simulink model "Full_RC_with_AVO"  (Simulink 8.3)
settings: Solver=ode1  StartTime=0.0  StopTime=500000.0  FixedStep=0.1  RelTol=1e-3
libraries: simulink x2
settings Model: Creator=user  LastModifiedBy=user
settings DataIOCC: SignalLoggingSaveFormat=Dataset
settings DebuggingCC: UnderspecifiedInitializationDetection=Simplified  StateNameClashWarn=none
settings GRTTargetCC: CombineOutputUpdateFcns=on  GRTInterface=off

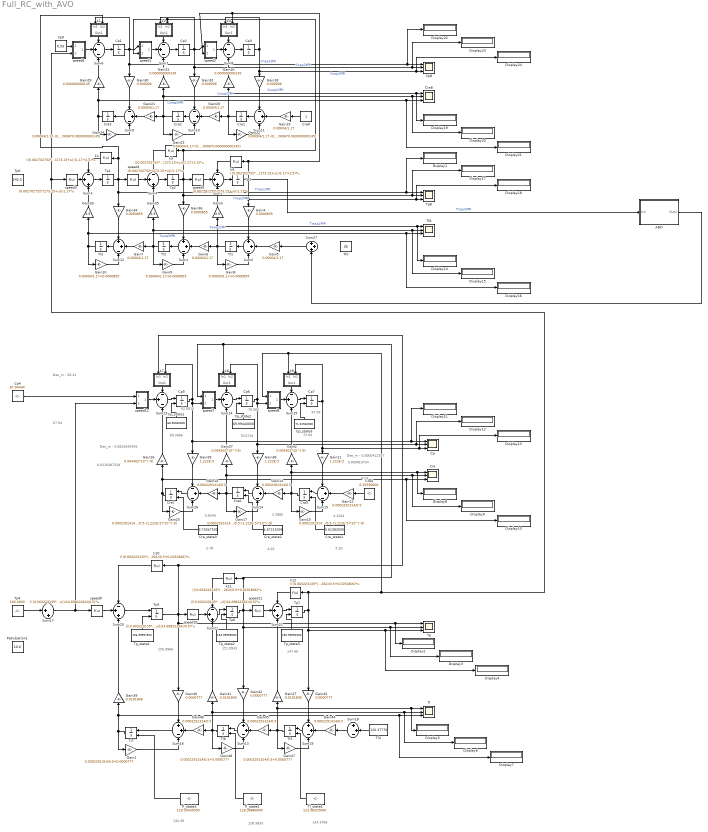
== system Full_RC_with_AVO ==
  note: Des_m - 0.0000412357
  note: Des_m - 0.0815645409
  note: 0.000010734
  note: 0.0216487318
  note: 0.9249
  note: 2.3980
  note: 4.2264
  note: 62.8910
  note: 78.085
  note: 97.09
  note: 67.94
  note: 2.78
  note: 4.02
  note: 5.26
  note: 72.04
  note: 70.6733
  note: 69.3066
  note: 132.39
  note: 128.3833
  note: 124.3766
  note: 147.99
  note: 151.9933
  note: 156.9966
  note: 4.24
  note: Des_m - 50.41
  Cp : Scope  NumInputPorts=3
      settings: TickLabels=on  ShowLegends=on  YMin=50~75~90  YMax=64~100~150  SaveName=CV_SM  DataFormat=Structure  SampleInput=on
  Cp0 : Constant  Value=0.53
  Cp1 : Integrator  InitialCondition=0.665
  Cp2 : Integrator  InitialCondition=0.803
  Cp3 : Integrator  InitialCondition=0.986
  Cp4 : Constant  Value=67.94440
  Cp5 : Integrator  InitialConditionSource=external  InitialCondition=69.3066
  Cp6 : Integrator  InitialConditionSource=external  InitialCondition=70.6733
  Cp7 : Integrator  InitialConditionSource=external  InitialCondition=72.04
  Cp8 : Scope  NumInputPorts=3
      settings: TickLabels=on  ShowLegends=on  YMin=50~75~90  YMax=64~100~150  SaveName=CV_SM1  DataFormat=Structure  SampleInput=on
  Cp_state1 : Constant  Value=68.96940000
  Cp_state2 : Constant  Value=69.99440000
  Cp_state3 : Constant  Value=71.01940000
  Cra : Scope  NumInputPorts=3
      settings: TickLabels=on  ShowLegends=on  YMin=4.17~2.4~0.84  YMax=4.28~2.5~1  SaveName=CF_SM  SampleInput=on
  Cra0 : Constant
  Cra1 : Integrator  InitialCondition=0.827
  Cra2 : Integrator  InitialCondition=0.6862
  Cra3 : Integrator  InitialCondition=0.5696
  Cra4 : Constant  Value=6.55550000
  Cra5 : Integrator  InitialConditionSource=external  InitialCondition=5.26
  Cra6 : Integrator  InitialConditionSource=external  InitialCondition=4.02
  Cra7 : Integrator  InitialConditionSource=external  InitialCondition=2.78
  Cra8 : Scope  NumInputPorts=3
      settings: TickLabels=on  ShowLegends=on  YMin=4.17~2.4~0.84  YMax=4.28~2.5~1  SaveName=CF_SM1  SampleInput=on
  Cra_state1 : Constant  Value=5.61382500
  Cra_state2 : Constant  Value=4.67215000
  Cra_state3 : Constant  Value=3.73047500
  Display{1..24} (24 alike) : Display
  Gain1 : Gain  Gain=0.0002291314/0.5+0.0000777
  Gain10 : Gain  Gain=0.00004/1.17+0.0000855
  Gain11 : Gain  Gain=1.222E-5
  Gain{12..14,44..46} (6 alike) : Gain  Gain=0.0002291314/0.5
  Gain15 : Gain  Gain=0.0002291314/0.5-(1.222E-5)*10^(-9)
  Gain16 : Gain  Gain=0.000000000145
  Gain17 : Gain  Gain=0.0002291314/0.5-(1.222E-5)*10^(-9)
  Gain18 : Gain  Gain=0.000006
  Gain{5..7,19..21} (6 alike) : Gain  Gain=0.00004/1.17
  Gain2 : Gain  Gain=0.004302*10^(-9)
  Gain22 : Gain  Gain=0.00004/1.17-(0.000006*0.000000000145)
  Gain23 : Gain  Gain=0.00004/1.17-(0.000006*0.000000000145)
  Gain24 : Gain  Gain=0.00004/1.17-(0.000006*0.000000000145)
  Gain25 : Gain  Gain=0.0002291314/0.5-(1.222E-5)*10^(-9)
  Gain26 : Gain  Gain=0.004302*10^(-9)
  Gain27 : Gain  Gain=0.0191806
  Gain28 : Gain  Gain=1.222E-5
  Gain29 : Gain  Gain=0.000000000145
  Gain3 : Gain  Gain=2.5
  Gain30 : Gain  Gain=0.000006
  Gain31 : Gain  Gain=0.000000000145
  Gain32 : Gain  Gain=0.000006
  Gain33 : Gain  Gain=2.5
  Gain34 : Gain  Gain=0.0000855
  Gain35 : Gain  Gain=2.5
  Gain36 : Gain  Gain=0.0000855
  Gain37 : Gain  Gain=0.004302*10^(-9)
  Gain38 : Gain  Gain=1.222E-5
  Gain39 : Gain  Gain=0.0191806
  Gain4 : Gain  Gain=0.0000855
  Gain40 : Gain  Gain=0.0000777
  Gain41 : Gain  Gain=0.0191806
  Gain42 : Gain  Gain=0.0000777
  Gain43 : Gain  Gain=0.0000777
  Gain47 : Gain  Gain=0.0002291314/0.5+0.0000777
  Gain48 : Gain  Gain=0.0002291314/0.5+0.0000777
  Gain8 : Gain  Gain=0.00004/1.17+0.0000855
  Gain9 : Gain  Gain=0.00004/1.17+0.0000855
  Petrubation1 : Constant  Value=10.0
  Sum{1..2,12..13,16,18..19} (7 alike) : Sum  Inputs=++-
  Sum{6..11,14..15,23..26} (12 alike) : Sum  Inputs=-+-
  Sum17 : Sum  Inputs=|++
  Sum{3..5,20..22} (6 alike) : Sum  Inputs=-++
  Sum27 : Sum  Inputs=+++
  Tl : Scope  NumInputPorts=3
      settings: TickLabels=on  ShowLegends=on  YMin=13~10~8.800000000000001  YMax=15.2~21~10.55  SaveName=TF_SM  SampleInput=on
  Tl0 : Constant  Value=30
  Tl1 : Integrator  InitialCondition=58.28
  Tl2 : Integrator  InitialCondition=86.23
  Tl3 : Integrator  InitialCondition=111.75
  Tl4 : Constant  Value=120.37770
  Tl5 : Integrator  InitialConditionSource=external  InitialCondition=124.3766
  Tl6 : Integrator  InitialConditionSource=external  InitialCondition=128.3833
  Tl7 : Integrator  InitialConditionSource=external  InitialCondition=132.39
  Tl8 : Scope  NumInputPorts=3
      settings: TickLabels=on  ShowLegends=on  YMin=13~10~8.800000000000001  YMax=15.2~21~10.55  SaveName=TF_SM1  SampleInput=on
  "Tl_state1 " : Constant  Value=123.38325000
  Tl_state2 : Constant  Value=126.38880000
  Tl_state3 : Constant  Value=129.39435000
  Tp : Scope  NumInputPorts=3
      settings: TickLabels=on  ShowLegends=on  YMin=155.5~145~146  YMax=158.5~152~154.5  SaveName=TV_SM  SampleInput=on
  Tp0 : Constant  Value=142.5
  Tp1 : Integrator  InitialCondition=121.956
  Tp2 : Integrator  InitialCondition=97.4
  Tp3 : Integrator  InitialCondition=69.6  IgnoreLimit=on
  Tp4 : Constant  Value=160.0000
  Tp5 : Integrator  InitialConditionSource=external  InitialCondition=156.9966
  Tp6 : Integrator  InitialConditionSource=external  InitialCondition=151.9933
  Tp7 : Integrator  InitialConditionSource=external  InitialCondition=147.99  IgnoreLimit=on
  Tp8 : Scope  NumInputPorts=3
      settings: TickLabels=on  ShowLegends=on  YMin=155.5~145~146  YMax=158.5~152~154.5  SaveName=TV_SM1  SampleInput=on
  Tp_state1 : Constant  Value=156.99997500
  Tp_state2 : Constant  Value=153.99995000
  Tp_state3 : Constant  Value=150.99992500
  k1 : Subsystem
  k10 : Fcn  Expr=(((0.003223135*(273+u))/24.69822264)/0.5+0.0191806)*u
  k11 : Fcn  Expr=(((0.003223135*(273+u))/24.69822264)/0.5+0.0191806)*u
  k12 : Fcn  Expr=(((0.003223135*(273+u))/24.69822264)/0.5+0.0191806)*u
  k2 : Subsystem
  k3 : Subsystem
  k4 : Fcn  Expr=((0.002702752*(273.15+u))/1.17+2.5)*u
  k5 : Fcn  Expr=((0.002702752*(273.15+u))/1.17+2.5)*u
  k6 : Fcn  Expr=((0.002702752*(273.15+u))/1.17+2.5)*u
  k7 : Subsystem
  k8 : Subsystem
  k9 : Subsystem
  speed1 : Subsystem
  speed10 : Fcn  Expr=(((0.003223135*(273+u))/24.69822264)/0.5)*u
  speed11 : Fcn  Expr=(((0.003223135*(273+u))/24.69822264)/0.5)*u
  speed12 : Subsystem
  speed2 : Subsystem
  speed3 : Fcn  Expr=(0.002702752*(273.15+u))/1.17*u
  speed4 : Fcn  Expr=(0.002702752*(273.15+u))/1.17*u
  speed5 : Fcn  Expr=(0.002702752*(273.15+u))/1.17*u
  speed6 : Subsystem
  speed7 : Subsystem
  speed8 : Subsystem
  speed9 : Fcn  Expr=(((0.003223135*(273+u))/24.69822264)/0.5)*u
  АВО : Subsystem
  wires:
  Sum6/1 -> Cp1/1
  speed1/1(Out1) -> Sum7/2
  Sum7/1 -> Cp2/1
  speed2/1(Out1) -> Sum8/2
  Sum8/1 -> Cp3/1
  Cp1/1 -> Cp8/1, Display22/1, Gain30/1, k1/1(In1), speed1/1(In1)  "Cпар1УРК"
  Cp2/1 -> Display23/1, Cp8/2, Gain32/1, speed2/1(In1), k2/1(In1)  "Cпар2УРК"
  Gain29/1 -> Sum6/3
  Cp3/1 -> Display24/1, Cp8/3, Gain18/1, k3/1(In1)  "Cпар3УРК"
  Gain31/1 -> Sum7/3
  Gain16/1 -> Sum8/3
  Gain30/1 -> Sum9/1
  Gain32/1 -> Sum10/1
  Gain18/1 -> Sum11/1
  Gain19/1 -> Sum11/2
  Sum11/1 -> Cra1/1
  Cra1/1 -> Gain22/1, Gain20/1, Display19/1, Cra8/1, Gain16/1  "Cжид1УРК"
  Gain20/1 -> Sum10/2
  Sum10/1 -> Cra2/1
  Cra2/1 -> Gain23/1, Gain21/1, Display20/1, Cra8/2, Gain31/1  "Cжид2УРК"
  Gain21/1 -> Sum9/2
  Sum9/1 -> Cra3/1
  Cra3/1 -> Gain24/1, Display21/1, Cra8/3, Gain29/1  "Cжид3УРК"
  Gain22/1 -> Sum11/3
  Gain23/1 -> Sum10/3
  Gain24/1 -> Sum9/3
  speed3/1 -> Sum3/2
  k4/1 -> Sum3/1
  Sum3/1 -> Tp1/1
  speed4/1 -> Sum4/2
  k5/1 -> Sum4/1
  Sum4/1 -> Tp2/1
  speed5/1 -> Sum5/2
  k6/1 -> Sum5/1
  Sum5/1 -> Tp3/1
  Tp1/1 -> Display1/1, Tp8/1, Gain34/1, k4/1, k1/2(In2), speed4/1  "Tпар1УРК"
  Gain33/1 -> Sum3/3
  Tp3/1 -> АВО/1(In1), Display18/1, Tp8/3, Gain4/1, k6/1, k3/2(In2), speed2/2(In2)  "Tпар3УРК"
  Gain35/1 -> Sum4/3
  Gain3/1 -> Sum5/3
  Gain34/1 -> Sum12/1
  Gain36/1 -> Sum1/1
  Gain4/1 -> Sum2/1
  Gain5/1 -> Sum2/2
  Sum2/1 -> Tl1/1
  Tl1/1 -> Gain8/1, Gain6/1, Display14/1, Tl8/1, Gain3/1  "Tжид1УРК"
  Gain6/1 -> Sum1/2
  Sum1/1 -> Tl2/1
  Tl2/1 -> Gain9/1, Gain7/1, Display15/1, Tl8/2, Gain35/1  "Tжид2УРК"
  Gain7/1 -> Sum12/2
  Sum12/1 -> Tl3/1
  Tl3/1 -> Gain10/1, Display16/1, Tl8/3, Gain33/1  "Tжид3УРК"
  Gain8/1 -> Sum2/3
  Gain9/1 -> Sum1/3
  Gain10/1 -> Sum12/3
  speed6/1(Out1) -> Sum6/2
  Cp0/1 -> speed6/1(In1)
  k1/1(Out1) -> Sum6/1
  k2/1(Out1) -> Sum7/1
  k3/1(Out1) -> Sum8/1
  Cra0/1 -> Gain19/1
  Sum23/1 -> Cp5/1
  speed7/1(Out1) -> Sum24/2
  Sum24/1 -> Cp6/1
  speed8/1(Out1) -> Sum25/2
  Sum25/1 -> Cp7/1
  Cp5/1 -> speed7/2(In2), Gain28/1, Cp/1, Display11/1, k7/2(In2)
  Gain26/1 -> Sum23/3
  Cp7/1 -> k9/2(In2), Gain11/1, Display13/1, Cp/3
  Gain37/1 -> Sum24/3
  Gain2/1 -> Sum25/3
  Gain28/1 -> Sum26/1
  Gain38/1 -> Sum14/1
  Gain11/1 -> Sum15/1
  Gain12/1 -> Sum15/2
  Sum15/1 -> Cra5/1
  Cra5/1 -> Gain15/1, Gain13/1, Gain2/1, Display8/1, Cra/1
  Gain13/1 -> Sum14/2
  Sum14/1 -> Cra6/1
  Gain14/1 -> Sum26/2
  Sum26/1 -> Cra7/1
  Gain15/1 -> Sum15/3
  Gain17/1 -> Sum14/3
  Gain25/1 -> Sum26/3
  speed9/1 -> Sum20/2
  k10/1 -> Sum20/1
  Sum20/1 -> Tp5/1
  speed10/1 -> Sum21/2
  k11/1 -> Sum21/1
  Sum21/1 -> Tp6/1
  speed11/1 -> Sum22/2
  k12/1 -> Sum22/1
  Sum22/1 -> Tp7/1
  Gain39/1 -> Sum20/3
  Gain41/1 -> Sum21/3
  Gain27/1 -> Sum22/3
  Gain40/1 -> Sum16/1
  Gain42/1 -> Sum13/1
  Gain43/1 -> Sum19/1
  Gain44/1 -> Sum19/2
  Sum19/1 -> Tl5/1
  Tl5/1 -> Gain47/1, Gain45/1, Gain27/1, Display5/1, Tl/1
  Gain45/1 -> Sum13/2
  Sum13/1 -> Tl6/1
  Gain46/1 -> Sum16/2
  Sum16/1 -> Tl7/1
  Gain47/1 -> Sum19/3
  Gain48/1 -> Sum13/3
  Gain1/1 -> Sum16/3
  speed12/1(Out1) -> Sum23/2
  Cp4/1 -> speed12/1(In1)
  k7/1(Out1) -> Sum23/1
  k8/1(Out1) -> Sum24/1
  k9/1(Out1) -> Sum25/1
  Cra4/1 -> Gain12/1
  Sum17/1 -> speed9/1, speed12/2(In2)
  Sum18/1 -> Gain44/1
  Tp4/1 -> Sum17/1
  Tl4/1 -> Sum18/2
  Tp6/1 -> Gain42/1, Display3/1, Tp/2, k11/1, speed7/1(In1), k8/1(In1), speed11/1
  Tp5/1 -> Gain40/1, Display2/1, Tp/1, k10/1, k7/1(In1), speed10/1
  Tp_state1/1 -> Tp5/2
  Tp_state3/1 -> Tp7/2
  "Tl_state1 "/1 -> Tl5/2
  Tl_state2/1 -> Tl6/2
  Tl_state3/1 -> Tl7/2
  Cp_state1/1 -> Cp5/2
  Cp_state2/1 -> Cp6/2
  Cp_state3/1 -> Cp7/2
  Cra_state1/1 -> Cra5/2
  Cra_state2/1 -> Cra6/2
  Cra_state3/1 -> Cra7/2
  Tp_state2/1 -> Tp6/2
  Tp7/1 -> Gain43/1, Display4/1, Tp/3, k12/1, k9/1(In1), speed8/1(In1), speed6/2(In2), speed3/1
  Tp2/1 -> Display17/1, Tp8/2, Gain36/1, k5/1, speed1/2(In2), k2/2(In2), speed5/1  "Tпар2УРК"
  Tl6/1 -> Gain48/1, Gain46/1, Gain41/1, Display6/1, Tl/2
  Tl7/1 -> Gain1/1, Gain39/1, Display7/1, Tl/3
  Cra6/1 -> Gain17/1, Gain14/1, Gain37/1, Display9/1, Cra/2
  Cra7/1 -> Gain25/1, Gain26/1, Display10/1, Cra/3
  Cp6/1 -> speed8/2(In2), Gain38/1, Display12/1, Cp/2, k8/2(In2)
  АВО/1(Out1) -> Sum27/3
  Sum27/1 -> Gain5/1

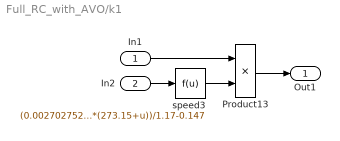
== system Full_RC_with_AVO/k1 ==
  In1 : Inport
  In2 : Inport  Port=2
  Product13 : Product  SaturateOnIntegerOverflow=on  InputSameDT=on  OutDataTypeStr=Inherit: Same as first input
  speed3 : Fcn  Expr=(0.002702752*(273.15+u))/1.17-0.147
  Out1 : Outport
  wires:
  Product13/1 -> Out1/1
  speed3/1 -> Product13/2
  In2/1 -> speed3/1
  In1/1 -> Product13/1

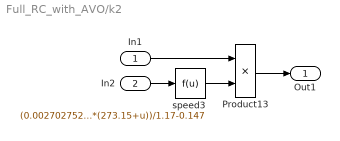
== system Full_RC_with_AVO/k2 ==
  In1 : Inport
  In2 : Inport  Port=2
  Product13 : Product  SaturateOnIntegerOverflow=on  InputSameDT=on  OutDataTypeStr=Inherit: Same as first input
  speed3 : Fcn  Expr=(0.002702752*(273.15+u))/1.17-0.147
  Out1 : Outport
  wires:
  In1/1 -> Product13/1
  In2/1 -> speed3/1
  speed3/1 -> Product13/2
  Product13/1 -> Out1/1

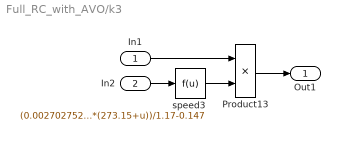
== system Full_RC_with_AVO/k3 ==
  In1 : Inport
  In2 : Inport  Port=2
  Product13 : Product  SaturateOnIntegerOverflow=on  InputSameDT=on  OutDataTypeStr=Inherit: Same as first input
  speed3 : Fcn  Expr=(0.002702752*(273.15+u))/1.17-0.147
  Out1 : Outport
  wires:
  Product13/1 -> Out1/1
  speed3/1 -> Product13/2
  In2/1 -> speed3/1
  In1/1 -> Product13/1

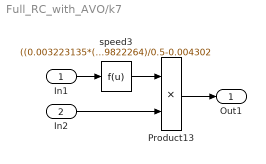
== system Full_RC_with_AVO/k7 ==
  In1 : Inport
  In2 : Inport  Port=2
  Product13 : Product  SaturateOnIntegerOverflow=on  InputSameDT=on  OutDataTypeStr=Inherit: Same as first input
  speed3 : Fcn  Expr=((0.003223135*(273+u))/24.69822264)/0.5-0.004302
  Out1 : Outport
  wires:
  Product13/1 -> Out1/1
  speed3/1 -> Product13/1
  In1/1 -> speed3/1
  In2/1 -> Product13/2

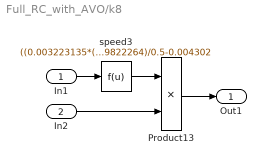
== system Full_RC_with_AVO/k8 ==
  In1 : Inport
  In2 : Inport  Port=2
  Product13 : Product  SaturateOnIntegerOverflow=on  InputSameDT=on  OutDataTypeStr=Inherit: Same as first input
  speed3 : Fcn  Expr=((0.003223135*(273+u))/24.69822264)/0.5-0.004302
  Out1 : Outport
  wires:
  Product13/1 -> Out1/1
  speed3/1 -> Product13/1
  In1/1 -> speed3/1
  In2/1 -> Product13/2

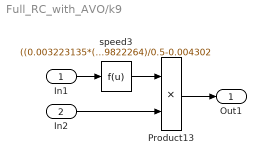
== system Full_RC_with_AVO/k9 ==
  In1 : Inport
  In2 : Inport  Port=2
  Product13 : Product  SaturateOnIntegerOverflow=on  InputSameDT=on  OutDataTypeStr=Inherit: Same as first input
  speed3 : Fcn  Expr=((0.003223135*(273+u))/24.69822264)/0.5-0.004302
  Out1 : Outport
  wires:
  Product13/1 -> Out1/1
  speed3/1 -> Product13/1
  In1/1 -> speed3/1
  In2/1 -> Product13/2

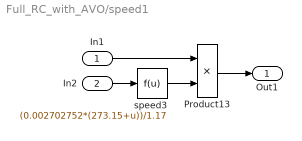
== system Full_RC_with_AVO/speed1 ==
  In1 : Inport
  In2 : Inport  Port=2
  Product13 : Product  SaturateOnIntegerOverflow=on  InputSameDT=on  OutDataTypeStr=Inherit: Same as first input
  speed3 : Fcn  Expr=(0.002702752*(273.15+u))/1.17
  Out1 : Outport
  wires:
  Product13/1 -> Out1/1
  speed3/1 -> Product13/2
  In2/1 -> speed3/1
  In1/1 -> Product13/1

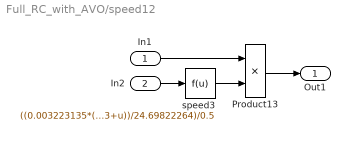
== system Full_RC_with_AVO/speed12 ==
  In1 : Inport
  In2 : Inport  Port=2
  Product13 : Product  SaturateOnIntegerOverflow=on  InputSameDT=on  OutDataTypeStr=Inherit: Same as first input
  speed3 : Fcn  Expr=((0.003223135*(273+u))/24.69822264)/0.5
  Out1 : Outport
  wires:
  In1/1 -> Product13/1
  In2/1 -> speed3/1
  speed3/1 -> Product13/2
  Product13/1 -> Out1/1

== system Full_RC_with_AVO/speed2 ==
  In1 : Inport
  In2 : Inport  Port=2
  Product13 : Product  SaturateOnIntegerOverflow=on  InputSameDT=on  OutDataTypeStr=Inherit: Same as first input
  speed3 : Fcn  Expr=(0.002702752*(273.15+u))/1.17
  Out1 : Outport
  wires:
  In1/1 -> Product13/1
  In2/1 -> speed3/1
  speed3/1 -> Product13/2
  Product13/1 -> Out1/1

== system Full_RC_with_AVO/speed6 ==
  In1 : Inport
  In2 : Inport  Port=2
  Product13 : Product  SaturateOnIntegerOverflow=on  InputSameDT=on  OutDataTypeStr=Inherit: Same as first input
  speed3 : Fcn  Expr=(0.002702752*(273.15+u))/1.17
  Out1 : Outport
  wires:
  In1/1 -> Product13/1
  In2/1 -> speed3/1
  speed3/1 -> Product13/2
  Product13/1 -> Out1/1

== system Full_RC_with_AVO/speed7 ==
  In1 : Inport
  In2 : Inport  Port=2
  Product13 : Product  SaturateOnIntegerOverflow=on  InputSameDT=on  OutDataTypeStr=Inherit: Same as first input
  speed3 : Fcn  Expr=((0.003223135*(273+u))/24.69822264)/0.5
  Out1 : Outport
  wires:
  Product13/1 -> Out1/1
  In2/1 -> Product13/2
  speed3/1 -> Product13/1
  In1/1 -> speed3/1

== system Full_RC_with_AVO/speed8 ==
  In1 : Inport
  In2 : Inport  Port=2
  Product13 : Product  SaturateOnIntegerOverflow=on  InputSameDT=on  OutDataTypeStr=Inherit: Same as first input
  speed3 : Fcn  Expr=((0.003223135*(273+u))/24.69822264)/0.5
  Out1 : Outport
  wires:
  Product13/1 -> Out1/1
  In2/1 -> Product13/2
  speed3/1 -> Product13/1
  In1/1 -> speed3/1

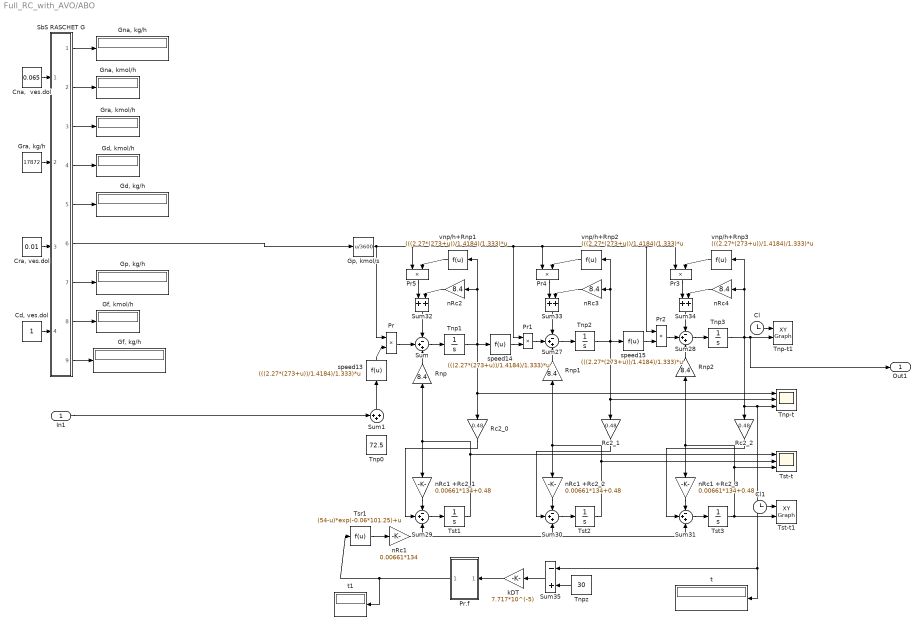
== system Full_RC_with_AVO/АВО ==
  In1 : Inport
  "Cd, ves.dol" : Constant
  Cl : Clock
  Cl1 : Clock
  "Cna,  ves.dol" : Constant  Value=0.065
  "Cra, ves.dol" : Constant  Value=0.01
  "Gd, kg/h" : Display
  "Gd, kmol/h" : Display
  "Gf, kg/h" : Display
  "Gf, kmol/h" : Display
  "Gna, kg/h" : Display
  "Gna, kmol/h" : Display
  "Gp, kmol/s" : Fcn  Expr=u/3600
  "Gp, kg/h" : Display
  "Gra, kg/h" : Constant  Value=17872
  "Gra, kmol/h" : Display
  Pr{,1..5} (6 alike) : Product  RndMeth=Zero
  Pr.f : Subsystem
  Rc2_0 : Gain  Gain=0.48
  Rc2_1 : Gain  Gain=0.48
  Rc2_2 : Gain  Gain=0.48
  Rnp : Gain  Gain=8.4
  Rnp1 : Gain  Gain=8.4
  Rnp2 : Gain  Gain=8.4
  SbS RASCHET G : Subsystem
  Sum{,27..31} (6 alike) : Sum  Inputs=-++
  Sum1 : Sum  Inputs=+++
  Sum32 : Sum
  Sum33 : Sum
  Sum34 : Sum
  Sum35 : Sum  Inputs=-+
  Tnp-t : Scope  NumInputPorts=3
      settings: YMin=67.9728~67.0823~66.2033  YMax=75.1278~74.1435~73.1721
  Tnp-t1 : simulink/Sinks/XY Graph  xmin=0  xmax=1000  ymin=10  ymax=50  st=-1
  Tnp0 : Constant  Value=72.5
  Tnp1 : Integrator  InitialCondition=55.042986606641151
  Tnp2 : Integrator  InitialCondition=42.494060413287038
  Tnp3 : Integrator  InitialCondition=33.818616670435347
  Tnpz : Constant  Value=30
  Tsr1 : Fcn  Expr=(54-u)*exp(-0.06*101.25)+u
  Tst-t : Scope  NumInputPorts=3
      settings: YMin=320.767~573.618~826.668  YMax=354.532~633.998~913.686
  Tst-t1 : simulink/Sinks/XY Graph  xmin=0  xmax=1000  ymin=10  ymax=50  st=-1
  Tst1 : Integrator  InitialCondition=30.749212884999000
  Tst2 : Integrator  InitialCondition=26.338794670104530
  Tst3 : Integrator  InitialCondition=23.289742144317184
  kDT : Gain  Gain=7.717*10^(-5)
  nRc1 : Gain  Gain=0.00661*134
  nRc1 +Rc2_1 : Gain  Gain=0.00661*134+0.48
  nRc1 +Rc2_2 : Gain  Gain=0.00661*134+0.48
  nRc1 +Rc2_3 : Gain  Gain=0.00661*134+0.48
  nRc2 : Gain  Gain=8.4
  nRc3 : Gain  Gain=8.4
  nRc4 : Gain  Gain=8.4
  speed13 : Fcn  Expr=(((2.27*(273+u))/1.4184)/1.333)*u
  speed14 : Fcn  Expr=(((2.27*(273+u))/1.4184)/1.333)*u
  speed15 : Fcn  Expr=(((2.27*(273+u))/1.4184)/1.333)*u
  t : Display
  t1 : Display
  vnp/h+Rnp1 : Fcn  Expr=(((2.27*(273+u))/1.4184)/1.333)*u
  vnp/h+Rnp2 : Fcn  Expr=(((2.27*(273+u))/1.4184)/1.333)*u
  vnp/h+Rnp3 : Fcn  Expr=(((2.27*(273+u))/1.4184)/1.333)*u
  Out1 : Outport
  wires:
  Sum/1 -> Tnp1/1
  Tnp2/1 -> speed15/1, Rc2_1/1, Tnp-t/2, vnp/h+Rnp2/1, nRc3/1
  Tnp1/1 -> speed14/1, Rc2_0/1, Tnp-t/1, vnp/h+Rnp1/1, nRc2/1
  Sum27/1 -> Tnp2/1
  Sum28/1 -> Tnp3/1
  vnp/h+Rnp3/1 -> Pr3/2
  vnp/h+Rnp2/1 -> Pr4/2
  vnp/h+Rnp1/1 -> Pr5/2
  Sum32/1 -> Sum/1
  Rnp2/1 -> Sum28/3
  Pr4/1 -> Sum33/1
  "Cra, ves.dol"/1 -> SbS RASCHET G/3(In3)
  Sum31/1 -> Tst3/1
  "Cd, ves.dol"/1 -> SbS RASCHET G/4(In4)
  Cl/1 -> Tnp-t1/1
  nRc1 +Rc2_1/1 -> Sum29/1
  Tst1/1 -> nRc1 +Rc2_1/1, Rnp/1, Tst-t/1
  "Gra, kg/h"/1 -> SbS RASCHET G/2(In2)
  SbS RASCHET G/1(Out1) -> "Gna, kg/h"/1
  SbS RASCHET G/5(Out5) -> "Gd, kg/h"/1
  Sum29/1 -> Tst1/1
  Pr/1 -> Sum/2
  Rc2_2/1 -> Sum31/2
  speed14/1 -> Pr1/2
  Rnp/1 -> Sum/3
  nRc1/1 -> Sum29/3, Sum31/3, Sum30/3
  "Gp, kmol/s"/1 -> Pr/1, Pr5/1, Pr2/1, Pr3/1, Pr4/1, Pr1/1
  Tnp3/1 -> vnp/h+Rnp3/1, nRc4/1, Out1/1, Tnp-t1/2, Rc2_2/1, Tnp-t/3, t/1, Sum35/1
  Tst3/1 -> Tst-t1/2, nRc1 +Rc2_3/1, Rnp2/1, Tst-t/3
  Sum30/1 -> Tst2/1
  Pr5/1 -> Sum32/1
  Rc2_1/1 -> Sum30/2
  nRc1 +Rc2_3/1 -> Sum31/1
  Pr2/1 -> Sum28/2
  nRc2/1 -> Sum32/2
  nRc3/1 -> Sum33/2
  "Cna,  ves.dol"/1 -> SbS RASCHET G/1(In1)
  speed15/1 -> Pr2/2
  Sum33/1 -> Sum27/1
  nRc4/1 -> Sum34/2
  Sum34/1 -> Sum28/1
  nRc1 +Rc2_2/1 -> Sum30/1
  Rnp1/1 -> Sum27/3
  Cl1/1 -> Tst-t1/1
  Pr1/1 -> Sum27/2
  Pr3/1 -> Sum34/1
  speed13/1 -> Pr/2
  Tst2/1 -> nRc1 +Rc2_2/1, Rnp1/1, Tst-t/2
  Rc2_0/1 -> Sum29/2
  SbS RASCHET G/7(Out7) -> "Gp, kg/h"/1
  SbS RASCHET G/6(Out6) -> "Gp, kmol/s"/1
  SbS RASCHET G/4(Out4) -> "Gd, kmol/h"/1
  Tsr1/1 -> nRc1/1
  SbS RASCHET G/2(Out2) -> "Gna, kmol/h"/1
  SbS RASCHET G/3(Out3) -> "Gra, kmol/h"/1
  Pr.f/1(Out1) -> t1/1, Tsr1/1
  SbS RASCHET G/9(Out9) -> "Gf, kg/h"/1
  Sum35/1 -> kDT/1
  Tnpz/1 -> Sum35/2
  kDT/1 -> Pr.f/1(In1)
  SbS RASCHET G/8(Out8) -> "Gf, kmol/h"/1
  Sum1/1 -> speed13/1
  In1/1 -> Sum1/1

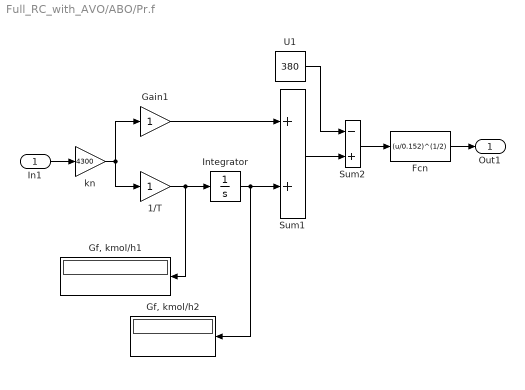
== system Full_RC_with_AVO/АВО/Pr.f ==
  In1 : Inport
  1/T : Gain
  Fcn : Fcn  Expr=(u/0.152)^(1/2)
  Gain1 : Gain
  "Gf, kmol/h1" : Display
  "Gf, kmol/h2" : Display
  Integrator : Integrator  InitialCondition=403.6
  Sum1 : Sum
  Sum2 : Sum  Inputs=-+
  U1 : Constant  Value=380
  kn : Gain  Gain=4300
  Out1 : Outport
  wires:
  kn/1 -> 1/T/1, Gain1/1
  1/T/1 -> Integrator/1, "Gf, kmol/h1"/1
  Integrator/1 -> Sum1/2, "Gf, kmol/h2"/1
  Gain1/1 -> Sum1/1
  Sum1/1 -> Sum2/2
  U1/1 -> Sum2/1
  In1/1 -> kn/1
  Fcn/1 -> Out1/1
  Sum2/1 -> Fcn/1

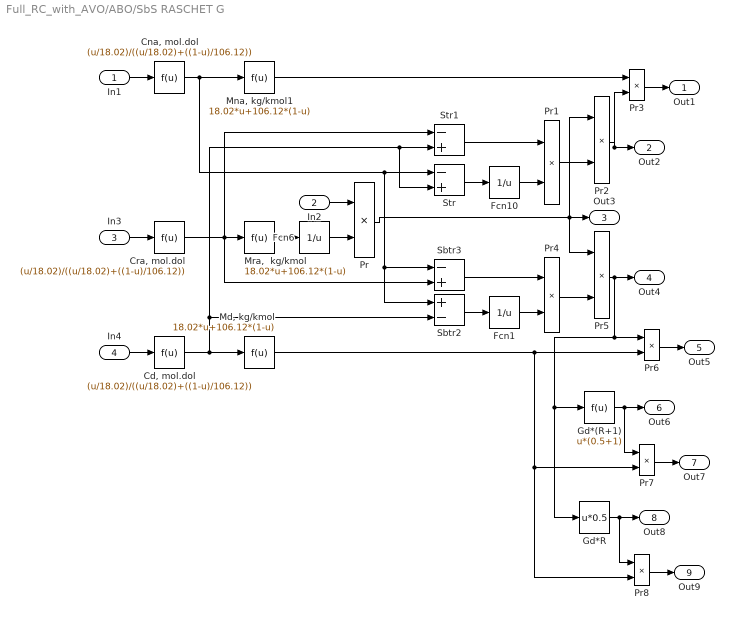
== system Full_RC_with_AVO/АВО/SbS RASCHET G ==
  In1 : Inport
  In2 : Inport  Port=2
  In3 : Inport  Port=3
  In4 : Inport  Port=4
  "Cd, mol.dol" : Fcn  Expr=(u/18.02)/((u/18.02)+((1-u)/106.12))
  "Cna, mol.dol" : Fcn  Expr=(u/18.02)/((u/18.02)+((1-u)/106.12))
  "Cra, mol.dol" : Fcn  Expr=(u/18.02)/((u/18.02)+((1-u)/106.12))
  Fcn1 : Fcn  Expr=1/u
  Fcn10 : Fcn  Expr=1/u
  Fcn6 : Fcn  Expr=1/u
  Gd*(R+1) : Fcn  Expr=u*(0.5+1)
  Gd*R : Fcn  Expr=u*0.5
  "Md, kg/kmol" : Fcn  Expr=18.02*u+106.12*(1-u)
  "Mna, kg/kmol1" : Fcn  Expr=18.02*u+106.12*(1-u)
  "Mra,  kg/kmol" : Fcn  Expr=18.02*u+106.12*(1-u)
  Pr{,1..8} (9 alike) : Product  RndMeth=Zero
  Sbtr2 : Sum  Inputs=+-
  Sbtr3 : Sum  Inputs=-+
  Str : Sum  Inputs=-+
  Str1 : Sum  Inputs=-+
  Out1 : Outport
  Out2 : Outport  Port=2
  Out3 : Outport  Port=3
  Out4 : Outport  Port=4
  Out5 : Outport  Port=5
  Out6 : Outport  Port=6
  Out7 : Outport  Port=7
  Out8 : Outport  Port=8
  Out9 : Outport  Port=9
  wires:
  "Mna, kg/kmol1"/1 -> Pr3/1
  "Cna, mol.dol"/1 -> "Mna, kg/kmol1"/1, Str/1, Sbtr3/1, Sbtr2/1
  "Cra, mol.dol"/1 -> "Mra,  kg/kmol"/1, Str1/1, Sbtr3/2
  "Cd, mol.dol"/1 -> "Md, kg/kmol"/1, Str1/2, Str/2, Sbtr2/2
  "Mra,  kg/kmol"/1 -> Fcn6/1
  Fcn6/1 -> Pr/2
  Pr/1 -> Pr2/1, Out3/1, Pr5/1
  Str/1 -> Fcn10/1
  Fcn10/1 -> Pr1/2
  Pr2/1 -> Pr3/2, Out2/1
  Pr1/1 -> Pr2/2
  Str1/1 -> Pr1/1
  Fcn1/1 -> Pr4/2
  Pr5/1 -> Pr6/1, Gd*(R+1)/1, Gd*R/1, Out4/1
  Pr4/1 -> Pr5/2
  "Md, kg/kmol"/1 -> Pr6/2, Pr7/2, Pr8/2
  Sbtr2/1 -> Fcn1/1
  Sbtr3/1 -> Pr4/1
  Gd*(R+1)/1 -> Pr7/1, Out6/1
  Gd*R/1 -> Pr8/1, Out8/1
  In1/1 -> "Cna, mol.dol"/1
  Pr3/1 -> Out1/1
  In2/1 -> Pr/1
  In3/1 -> "Cra, mol.dol"/1
  Pr6/1 -> Out5/1
  In4/1 -> "Cd, mol.dol"/1
  Pr7/1 -> Out7/1
  Pr8/1 -> Out9/1
